simulink library "roller485lib"  (R2023a)
settings: Solver=VariableStepAuto  StartTime=0.0  StopTime=10.0  RelTol=1e-3
libraries: arduinolib x106, simulink x45
(part 2 of 3)

== system roller485lib/Basic I2C Write/position PID ==
  " x 10^5 " : Gain  Gain=1e5
  D : Constant  Value=position_D
  Data Type Conversion1 : DataTypeConversion  OutDataTypeStr=uint32  SaturateOnIntegerOverflow=off  RndMeth=Floor
  Data Type Conversion2 : DataTypeConversion  OutDataTypeStr=uint32  SaturateOnIntegerOverflow=off  RndMeth=Floor
  Data Type Conversion3 : DataTypeConversion  OutDataTypeStr=uint32  SaturateOnIntegerOverflow=off  RndMeth=Floor
  I : Constant  Value=position_I
  I2C Write (0xA0) : arduinolib/I2C Write  I2CModule=0  Mode=Master  SlaveAddress=I2CAddress  SlaveByteOrder=LittleEndian  Direction=Transmitter  RegisterAddressMode=on  RegisterAddress=0xA0  SlaveDataType=uint8  DataLength=1  NoAck=off  RepeatedStart=off  OutputStatus=off  blockPlatform=ARDUINO
  I2C Write (0xA4) : arduinolib/I2C Write  I2CModule=0  Mode=Master  SlaveAddress=I2CAddress  SlaveByteOrder=LittleEndian  Direction=Transmitter  RegisterAddressMode=on  RegisterAddress=0xA4  SlaveDataType=uint8  DataLength=1  NoAck=off  RepeatedStart=off  OutputStatus=off  blockPlatform=ARDUINO
  I2C Write (0xA8) : arduinolib/I2C Write  I2CModule=0  Mode=Master  SlaveAddress=I2CAddress  SlaveByteOrder=LittleEndian  Direction=Transmitter  RegisterAddressMode=on  RegisterAddress=0xA8  SlaveDataType=uint8  DataLength=1  NoAck=off  RepeatedStart=off  OutputStatus=off  blockPlatform=ARDUINO
  P : Constant  Value=position_P
  x 10^5 : Gain  Gain=1e5
  x 10^7 : Gain  Gain=1e7
  wires:
  P/1 -> x 10^5/1
  I/1 -> x 10^7/1
  D/1 -> " x 10^5 "/1
  Data Type Conversion1/1 -> I2C Write (0xA0)/1
  Data Type Conversion3/1 -> I2C Write (0xA8)/1
  Data Type Conversion2/1 -> I2C Write (0xA4)/1
  x 10^5/1 -> Data Type Conversion1/1
  x 10^7/1 -> Data Type Conversion2/1
  " x 10^5 "/1 -> Data Type Conversion3/1

== system roller485lib/Basic I2C Write/position PID (within set time) ==
  Clock : Clock
  Compare To Constant : simulink/Logic and Bit Operations/Compare To Constant  relop=<=  const=set_time  OutDataTypeStr=boolean
  D : Constant  Value=position_D
  Enabled Subsystem : Subsystem  TreatAsAtomicUnit=on
  I : Constant  Value=position_I
  P : Constant  Value=position_P
  wires:
  D/1 -> Enabled Subsystem/3(D)
  I/1 -> Enabled Subsystem/2(I)
  P/1 -> Enabled Subsystem/1(P)
  Compare To Constant/1 -> Enabled Subsystem/Enable
  Clock/1 -> Compare To Constant/1

== system roller485lib/Basic I2C Write/speed PID ==
  " x 10^5 " : Gain  Gain=1e5
  D : Constant  Value=speed_D
  Data Type Conversion2 : DataTypeConversion  OutDataTypeStr=uint32  SaturateOnIntegerOverflow=off  RndMeth=Floor
  Data Type Conversion4 : DataTypeConversion  OutDataTypeStr=uint32  SaturateOnIntegerOverflow=off  RndMeth=Floor
  Data Type Conversion6 : DataTypeConversion  OutDataTypeStr=uint32  SaturateOnIntegerOverflow=off  RndMeth=Floor
  I : Constant  Value=speed_I
  I2C Write (0x70) : arduinolib/I2C Write  I2CModule=0  Mode=Master  SlaveAddress=I2CAddress  SlaveByteOrder=LittleEndian  Direction=Transmitter  RegisterAddressMode=on  RegisterAddress=0x70  SlaveDataType=uint8  DataLength=1  NoAck=off  RepeatedStart=off  OutputStatus=off  blockPlatform=ARDUINO
  I2C Write (0x74) : arduinolib/I2C Write  I2CModule=0  Mode=Master  SlaveAddress=I2CAddress  SlaveByteOrder=LittleEndian  Direction=Transmitter  RegisterAddressMode=on  RegisterAddress=0x74  SlaveDataType=uint8  DataLength=1  NoAck=off  RepeatedStart=off  OutputStatus=off  blockPlatform=ARDUINO
  I2C Write (0x78) : arduinolib/I2C Write  I2CModule=0  Mode=Master  SlaveAddress=I2CAddress  SlaveByteOrder=LittleEndian  Direction=Transmitter  RegisterAddressMode=on  RegisterAddress=0x78  SlaveDataType=uint8  DataLength=1  NoAck=off  RepeatedStart=off  OutputStatus=off  blockPlatform=ARDUINO
  P : Constant  Value=speed_P
  x 10^5 : Gain  Gain=1e5
  x 10^7 : Gain  Gain=1e7
  wires:
  D/1 -> " x 10^5 "/1
  I/1 -> x 10^7/1
  P/1 -> x 10^5/1
  Data Type Conversion2/1 -> I2C Write (0x70)/1
  Data Type Conversion4/1 -> I2C Write (0x74)/1
  Data Type Conversion6/1 -> I2C Write (0x78)/1
  x 10^5/1 -> Data Type Conversion2/1
  x 10^7/1 -> Data Type Conversion4/1
  " x 10^5 "/1 -> Data Type Conversion6/1

== system roller485lib/Basic I2C Write/speed PID (within set time) ==
  Clock : Clock
  Compare To Constant : simulink/Logic and Bit Operations/Compare To Constant  relop=<=  const=set_time  OutDataTypeStr=boolean
  D : Constant  Value=speed_D
  Enabled Subsystem : Subsystem  TreatAsAtomicUnit=on
  I : Constant  Value=speed_I
  P : Constant  Value=speed_P
  wires:
  Clock/1 -> Compare To Constant/1
  Compare To Constant/1 -> Enabled Subsystem/Enable
  P/1 -> Enabled Subsystem/1(P)
  I/1 -> Enabled Subsystem/2(I)
  D/1 -> Enabled Subsystem/3(D)

== system roller485lib/I2C Read/absolute angle detection [deg] ==
  Data Type Conversion : DataTypeConversion  OutDataTypeStr=double  SaturateOnIntegerOverflow=off  RndMeth=Floor
  I2C Read (0x90) : arduinolib/I2C Read  I2CModule=0  Mode=Master  SlaveAddress=I2CAddress  SlaveByteOrder=LittleEndian  Direction=Receiver  RegisterAddressMode=on  RegisterAddress=0x90  SlaveDataType=int32  DataLength=1  NoAck=off  RepeatedStart=off  OutputStatus=off  blockPlatform=ARDUINO  SampleTime=sample_time
  Reshape : Reshape
  x (1/100) : Gain  Gain=1/100
  deg : Outport
  wires:
  x (1/100)/1 -> Reshape/1
  I2C Read (0x90)/1 -> Data Type Conversion/1
  Data Type Conversion/1 -> x (1/100)/1
  Reshape/1 -> deg/1

== system roller485lib/I2C Read/absolute angle detection [rad] ==
  Data Type Conversion : DataTypeConversion  OutDataTypeStr=double  SaturateOnIntegerOverflow=off  RndMeth=Floor
  I2C Read (0x90) : arduinolib/I2C Read  I2CModule=0  Mode=Master  SlaveAddress=I2CAddress  SlaveByteOrder=LittleEndian  Direction=Receiver  RegisterAddressMode=on  RegisterAddress=0x90  SlaveDataType=int32  DataLength=1  NoAck=off  RepeatedStart=off  OutputStatus=off  blockPlatform=ARDUINO  SampleTime=sample_time
  Reshape : Reshape
  deg to rad : Gain  Gain=pi/180
  x (1/100) : Gain  Gain=1/100
  rad : Outport
  wires:
  x (1/100)/1 -> deg to rad/1
  deg to rad/1 -> Reshape/1
  Data Type Conversion/1 -> x (1/100)/1
  I2C Read (0x90)/1 -> Data Type Conversion/1
  Reshape/1 -> rad/1

== system roller485lib/I2C Read/angular velocity detection using LPF [rad//s] ==
  Data Type Conversion : DataTypeConversion  OutDataTypeStr=double  SaturateOnIntegerOverflow=off  RndMeth=Floor
  I2C Read (0x60) : arduinolib/I2C Read  I2CModule=0  Mode=Master  SlaveAddress=I2CAddress  SlaveByteOrder=LittleEndian  Direction=Receiver  RegisterAddressMode=on  RegisterAddress=0x60  SlaveDataType=int32  DataLength=1  NoAck=off  RepeatedStart=off  OutputStatus=off  blockPlatform=ARDUINO  SampleTime=sample_time
  Reshape : Reshape
  rpm to rad/s : Gain  Gain=2*pi/60
  x (1/100) : Gain  Gain=1/100
  rad/s : Outport
  wires:
  x (1/100)/1 -> rpm to rad/s/1
  rpm to rad/s/1 -> Reshape/1
  I2C Read (0x60)/1 -> Data Type Conversion/1
  Data Type Conversion/1 -> x (1/100)/1
  Reshape/1 -> rad/s/1

== system roller485lib/I2C Read/angular velocity detection using LPF [rpm] ==
  Data Type Conversion : DataTypeConversion  OutDataTypeStr=double  SaturateOnIntegerOverflow=off  RndMeth=Floor
  I2C Read (0x60) : arduinolib/I2C Read  I2CModule=0  Mode=Master  SlaveAddress=I2CAddress  SlaveByteOrder=LittleEndian  Direction=Receiver  RegisterAddressMode=on  RegisterAddress=0x60  SlaveDataType=int32  DataLength=1  NoAck=off  RepeatedStart=off  OutputStatus=off  blockPlatform=ARDUINO  SampleTime=sample_time
  Reshape : Reshape
  x (1/100) : Gain  Gain=1/100
  rpm : Outport
  wires:
  x (1/100)/1 -> Reshape/1
  Data Type Conversion/1 -> x (1/100)/1
  I2C Read (0x60)/1 -> Data Type Conversion/1
  Reshape/1 -> rpm/1

== system roller485lib/I2C Read/current detection [A] ==
  Data Type Conversion : DataTypeConversion  OutDataTypeStr=double  SaturateOnIntegerOverflow=off  RndMeth=Floor
  I2C Read (0xC0) : arduinolib/I2C Read  I2CModule=0  Mode=Master  SlaveAddress=I2CAddress  SlaveByteOrder=LittleEndian  Direction=Receiver  RegisterAddressMode=on  RegisterAddress=0xC0  SlaveDataType=int32  DataLength=1  NoAck=off  RepeatedStart=off  OutputStatus=off  blockPlatform=ARDUINO  SampleTime=sample_time
  Reshape : Reshape
  mA to A : Gain  Gain=1/1000
  x (1/100) : Gain  Gain=1/100
  A : Outport
  wires:
  x (1/100)/1 -> mA to A/1
  Data Type Conversion/1 -> x (1/100)/1
  mA to A/1 -> Reshape/1
  I2C Read (0xC0)/1 -> Data Type Conversion/1
  Reshape/1 -> A/1

== system roller485lib/I2C Read/current detection [mA] ==
  Data Type Conversion : DataTypeConversion  OutDataTypeStr=double  SaturateOnIntegerOverflow=off  RndMeth=Floor
  I2C Read (0xC0) : arduinolib/I2C Read  I2CModule=0  Mode=Master  SlaveAddress=I2CAddress  SlaveByteOrder=LittleEndian  Direction=Receiver  RegisterAddressMode=on  RegisterAddress=0xC0  SlaveDataType=int32  DataLength=1  NoAck=off  RepeatedStart=off  OutputStatus=off  blockPlatform=ARDUINO  SampleTime=sample_time
  Reshape : Reshape
  x (1/100) : Gain  Gain=1/100
  mA : Outport
  wires:
  Data Type Conversion/1 -> x (1/100)/1
  x (1/100)/1 -> Reshape/1
  I2C Read (0xC0)/1 -> Data Type Conversion/1
  Reshape/1 -> mA/1

== system roller485lib/I2C Read/relative angle detection [deg] ==
  Clock : Clock
  Compare To Constant : simulink/Logic and Bit Operations/Compare To Constant  relop=<=  const=set_time  OutDataTypeStr=boolean
  Data Type Conversion : DataTypeConversion  OutDataTypeStr=double  SaturateOnIntegerOverflow=off  RndMeth=Floor
  Enabled Subsystem (initialization of angle) : Subsystem  TreatAsAtomicUnit=on
  I2C Read (0x90) : arduinolib/I2C Read  I2CModule=0  Mode=Master  SlaveAddress=I2CAddress  SlaveByteOrder=LittleEndian  Direction=Receiver  RegisterAddressMode=on  RegisterAddress=0x90  SlaveDataType=int32  DataLength=1  NoAck=off  RepeatedStart=off  OutputStatus=off  blockPlatform=ARDUINO  SampleTime=sample_time
  Reshape : Reshape
  Sum : Sum  Inputs=-+|
  x (1/100) : Gain  Gain=1/100
  deg : Outport
  wires:
  Sum/1 -> x (1/100)/1
  Enabled Subsystem (initialization of angle)/1(phim(0)) -> Sum/1
  Data Type Conversion/1 -> Sum/2, Enabled Subsystem (initialization of angle)/1(phim)
  Clock/1 -> Compare To Constant/1
  x (1/100)/1 -> Reshape/1
  I2C Read (0x90)/1 -> Data Type Conversion/1
  Reshape/1 -> deg/1
  Compare To Constant/1 -> Enabled Subsystem (initialization of angle)/Enable

== system roller485lib/I2C Read/relative angle detection [rad] ==
  Clock : Clock
  Compare To Constant : simulink/Logic and Bit Operations/Compare To Constant  relop=<=  const=set_time  OutDataTypeStr=boolean
  Data Type Conversion : DataTypeConversion  OutDataTypeStr=double  SaturateOnIntegerOverflow=off  RndMeth=Floor
  Enabled Subsystem (initialization of angle) : Subsystem  TreatAsAtomicUnit=on
  I2C Read (0x90) : arduinolib/I2C Read  I2CModule=0  Mode=Master  SlaveAddress=I2CAddress  SlaveByteOrder=LittleEndian  Direction=Receiver  RegisterAddressMode=on  RegisterAddress=0x90  SlaveDataType=int32  DataLength=1  NoAck=off  RepeatedStart=off  OutputStatus=off  blockPlatform=ARDUINO  SampleTime=sample_time
  Reshape : Reshape
  Sum : Sum  Inputs=-+|
  deg to rad : Gain  Gain=pi/180
  x (1/100) : Gain  Gain=1/100
  rad : Outport
  wires:
  x (1/100)/1 -> deg to rad/1
  Clock/1 -> Compare To Constant/1
  Data Type Conversion/1 -> Enabled Subsystem (initialization of angle)/1(phim), Sum/2
  Enabled Subsystem (initialization of angle)/1(phim(0)) -> Sum/1
  Sum/1 -> x (1/100)/1
  deg to rad/1 -> Reshape/1
  I2C Read (0x90)/1 -> Data Type Conversion/1
  Reshape/1 -> rad/1
  Compare To Constant/1 -> Enabled Subsystem (initialization of angle)/Enable

== system roller485lib/I2C Write/absolute angle command [deg] ==
  command [deg] : Inport
  Clock1 : Clock
  Clock2 : Clock
  Compare To Constant1 : simulink/Logic and Bit Operations/Compare To Constant  relop=<=  const=set_time1  OutDataTypeStr=boolean
  Compare To Constant2 : simulink/Logic and Bit Operations/Compare To Constant  relop=<=  const=set_time2  OutDataTypeStr=boolean
  D : Constant  Value=position_D
  Data Type Conversion : DataTypeConversion  OutDataTypeStr=uint32  SaturateOnIntegerOverflow=off  RndMeth=Floor
  Enabled Subsystem (PID setting) : Subsystem  TreatAsAtomicUnit=on
  Enabled Subsystem (mode setting) : Subsystem  TreatAsAtomicUnit=on
  I : Constant  Value=position_I
  I2C Write (0x80) : arduinolib/I2C Write  I2CModule=0  Mode=Master  SlaveAddress=I2CAddress  SlaveByteOrder=LittleEndian  Direction=Transmitter  RegisterAddressMode=on  RegisterAddress=0x80  SlaveDataType=uint8  DataLength=1  NoAck=off  RepeatedStart=off  OutputStatus=off  blockPlatform=ARDUINO
  P : Constant  Value=position_P
  position mode : Constant  Value=2
  x 100 : Gain  Gain=100
  wires:
  P/1 -> Enabled Subsystem (PID setting)/1(P)
  Clock1/1 -> Compare To Constant1/1
  position mode/1 -> Enabled Subsystem (mode setting)/1(mode)
  I/1 -> Enabled Subsystem (PID setting)/2(I)
  x 100/1 -> Data Type Conversion/1
  D/1 -> Enabled Subsystem (PID setting)/3(D)
  Compare To Constant2/1 -> Enabled Subsystem (PID setting)/Enable
  Compare To Constant1/1 -> Enabled Subsystem (mode setting)/Enable
  Clock2/1 -> Compare To Constant2/1
  Data Type Conversion/1 -> I2C Write (0x80)/1
  command [deg]/1 -> x 100/1

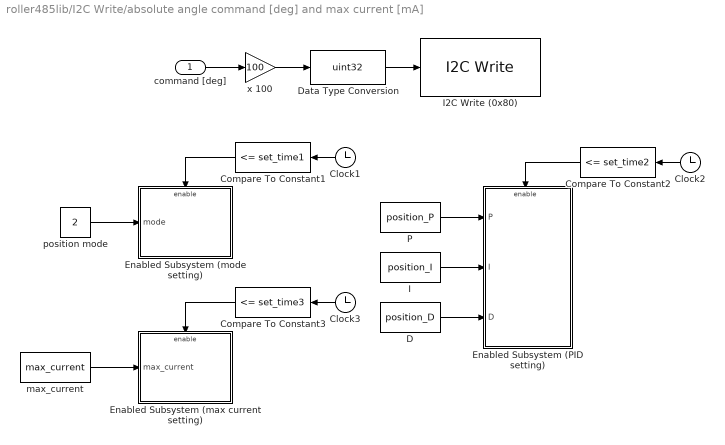
== system roller485lib/I2C Write/absolute angle command [deg] and max current [mA] ==
  command [deg] : Inport
  Clock1 : Clock
  Clock2 : Clock
  Clock3 : Clock
  Compare To Constant1 : simulink/Logic and Bit Operations/Compare To Constant  relop=<=  const=set_time1  OutDataTypeStr=boolean
  Compare To Constant2 : simulink/Logic and Bit Operations/Compare To Constant  relop=<=  const=set_time2  OutDataTypeStr=boolean
  Compare To Constant3 : simulink/Logic and Bit Operations/Compare To Constant  relop=<=  const=set_time3  OutDataTypeStr=boolean
  D : Constant  Value=position_D
  Data Type Conversion : DataTypeConversion  OutDataTypeStr=uint32  SaturateOnIntegerOverflow=off  RndMeth=Floor
  Enabled Subsystem (PID setting) : Subsystem  TreatAsAtomicUnit=on
  Enabled Subsystem (max current setting) : Subsystem  TreatAsAtomicUnit=on
  Enabled Subsystem (mode setting) : Subsystem  TreatAsAtomicUnit=on
  I : Constant  Value=position_I
  I2C Write (0x80) : arduinolib/I2C Write  I2CModule=0  Mode=Master  SlaveAddress=I2CAddress  SlaveByteOrder=LittleEndian  Direction=Transmitter  RegisterAddressMode=on  RegisterAddress=0x80  SlaveDataType=uint8  DataLength=1  NoAck=off  RepeatedStart=off  OutputStatus=off  blockPlatform=ARDUINO
  P : Constant  Value=position_P
  max_current : Constant  Value=max_current
  position mode : Constant  Value=2
  x 100 : Gain  Gain=100
  wires:
  P/1 -> Enabled Subsystem (PID setting)/1(P)
  Clock1/1 -> Compare To Constant1/1
  position mode/1 -> Enabled Subsystem (mode setting)/1(mode)
  I/1 -> Enabled Subsystem (PID setting)/2(I)
  Clock3/1 -> Compare To Constant3/1
  x 100/1 -> Data Type Conversion/1
  Compare To Constant3/1 -> Enabled Subsystem (max current setting)/Enable
  D/1 -> Enabled Subsystem (PID setting)/3(D)
  Compare To Constant2/1 -> Enabled Subsystem (PID setting)/Enable
  Compare To Constant1/1 -> Enabled Subsystem (mode setting)/Enable
  Clock2/1 -> Compare To Constant2/1
  max_current/1 -> Enabled Subsystem (max current setting)/1(max_current)
  Data Type Conversion/1 -> I2C Write (0x80)/1
  command [deg]/1 -> x 100/1

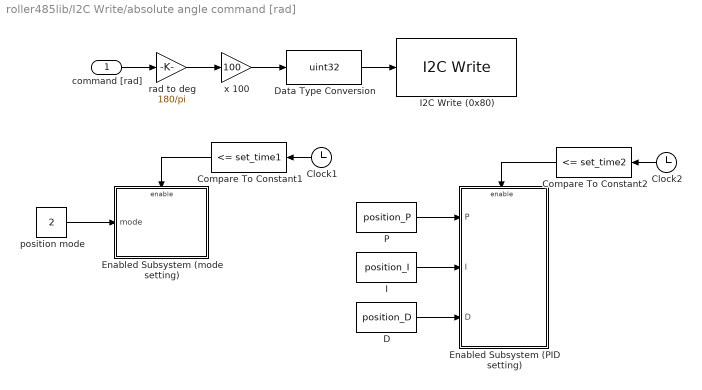
== system roller485lib/I2C Write/absolute angle command [rad] ==
  command [rad] : Inport
  Clock1 : Clock
  Clock2 : Clock
  Compare To Constant1 : simulink/Logic and Bit Operations/Compare To Constant  relop=<=  const=set_time1  OutDataTypeStr=boolean
  Compare To Constant2 : simulink/Logic and Bit Operations/Compare To Constant  relop=<=  const=set_time2  OutDataTypeStr=boolean
  D : Constant  Value=position_D
  Data Type Conversion : DataTypeConversion  OutDataTypeStr=uint32  SaturateOnIntegerOverflow=off  RndMeth=Floor
  Enabled Subsystem (PID setting) : Subsystem  TreatAsAtomicUnit=on
  Enabled Subsystem (mode setting) : Subsystem  TreatAsAtomicUnit=on
  I : Constant  Value=position_I
  I2C Write (0x80) : arduinolib/I2C Write  I2CModule=0  Mode=Master  SlaveAddress=I2CAddress  SlaveByteOrder=LittleEndian  Direction=Transmitter  RegisterAddressMode=on  RegisterAddress=0x80  SlaveDataType=uint8  DataLength=1  NoAck=off  RepeatedStart=off  OutputStatus=off  blockPlatform=ARDUINO
  P : Constant  Value=position_P
  position mode : Constant  Value=2
  rad to deg : Gain  Gain=180/pi
  x 100 : Gain  Gain=100
  wires:
  P/1 -> Enabled Subsystem (PID setting)/1(P)
  Clock1/1 -> Compare To Constant1/1
  position mode/1 -> Enabled Subsystem (mode setting)/1(mode)
  I/1 -> Enabled Subsystem (PID setting)/2(I)
  x 100/1 -> Data Type Conversion/1
  command [rad]/1 -> rad to deg/1
  D/1 -> Enabled Subsystem (PID setting)/3(D)
  Compare To Constant2/1 -> Enabled Subsystem (PID setting)/Enable
  Compare To Constant1/1 -> Enabled Subsystem (mode setting)/Enable
  Clock2/1 -> Compare To Constant2/1
  Data Type Conversion/1 -> I2C Write (0x80)/1
  rad to deg/1 -> x 100/1

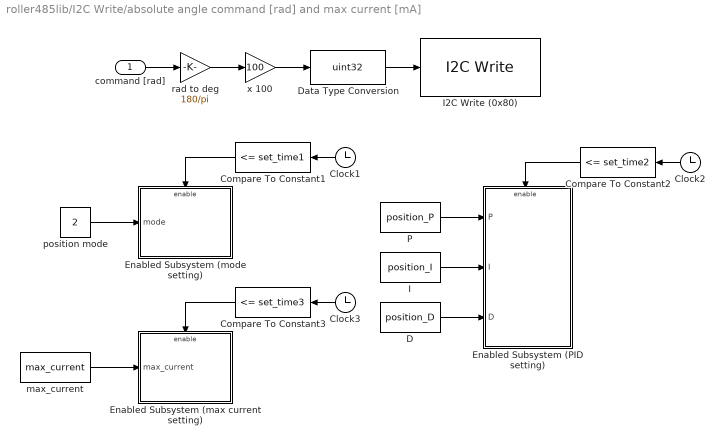
== system roller485lib/I2C Write/absolute angle command [rad] and max current [mA] ==
  command [rad] : Inport
  Clock1 : Clock
  Clock2 : Clock
  Clock3 : Clock
  Compare To Constant1 : simulink/Logic and Bit Operations/Compare To Constant  relop=<=  const=set_time1  OutDataTypeStr=boolean
  Compare To Constant2 : simulink/Logic and Bit Operations/Compare To Constant  relop=<=  const=set_time2  OutDataTypeStr=boolean
  Compare To Constant3 : simulink/Logic and Bit Operations/Compare To Constant  relop=<=  const=set_time3  OutDataTypeStr=boolean
  D : Constant  Value=position_D
  Data Type Conversion : DataTypeConversion  OutDataTypeStr=uint32  SaturateOnIntegerOverflow=off  RndMeth=Floor
  Enabled Subsystem (PID setting) : Subsystem  TreatAsAtomicUnit=on
  Enabled Subsystem (max current setting) : Subsystem  TreatAsAtomicUnit=on
  Enabled Subsystem (mode setting) : Subsystem  TreatAsAtomicUnit=on
  I : Constant  Value=position_I
  I2C Write (0x80) : arduinolib/I2C Write  I2CModule=0  Mode=Master  SlaveAddress=I2CAddress  SlaveByteOrder=LittleEndian  Direction=Transmitter  RegisterAddressMode=on  RegisterAddress=0x80  SlaveDataType=uint8  DataLength=1  NoAck=off  RepeatedStart=off  OutputStatus=off  blockPlatform=ARDUINO
  P : Constant  Value=position_P
  max_current : Constant  Value=max_current
  position mode : Constant  Value=2
  rad to deg : Gain  Gain=180/pi
  x 100 : Gain  Gain=100
  wires:
  command [rad]/1 -> rad to deg/1
  rad to deg/1 -> x 100/1
  Data Type Conversion/1 -> I2C Write (0x80)/1
  x 100/1 -> Data Type Conversion/1
  P/1 -> Enabled Subsystem (PID setting)/1(P)
  Clock1/1 -> Compare To Constant1/1
  Compare To Constant2/1 -> Enabled Subsystem (PID setting)/Enable
  I/1 -> Enabled Subsystem (PID setting)/2(I)
  D/1 -> Enabled Subsystem (PID setting)/3(D)
  Compare To Constant3/1 -> Enabled Subsystem (max current setting)/Enable
  Clock3/1 -> Compare To Constant3/1
  position mode/1 -> Enabled Subsystem (mode setting)/1(mode)
  max_current/1 -> Enabled Subsystem (max current setting)/1(max_current)
  Compare To Constant1/1 -> Enabled Subsystem (mode setting)/Enable
  Clock2/1 -> Compare To Constant2/1

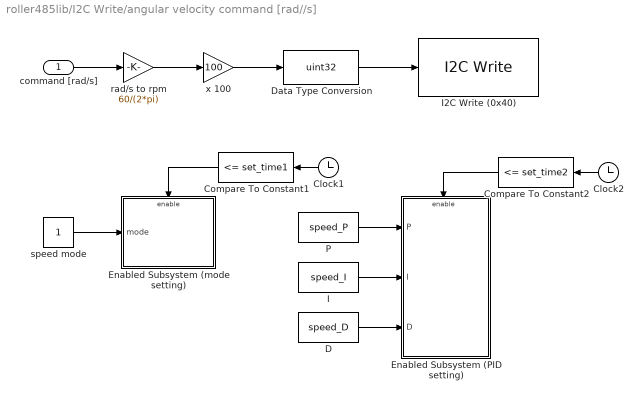
== system roller485lib/I2C Write/angular velocity command [rad//s] ==
  command [rad/s] : Inport
  Clock1 : Clock
  Clock2 : Clock
  Compare To Constant1 : simulink/Logic and Bit Operations/Compare To Constant  relop=<=  const=set_time1  OutDataTypeStr=boolean
  Compare To Constant2 : simulink/Logic and Bit Operations/Compare To Constant  relop=<=  const=set_time2  OutDataTypeStr=boolean
  D : Constant  Value=speed_D
  Data Type Conversion : DataTypeConversion  OutDataTypeStr=uint32  SaturateOnIntegerOverflow=off  RndMeth=Floor
  Enabled Subsystem (PID setting) : Subsystem  TreatAsAtomicUnit=on
  Enabled Subsystem (mode setting) : Subsystem  TreatAsAtomicUnit=on
  I : Constant  Value=speed_I
  I2C Write (0x40) : arduinolib/I2C Write  I2CModule=0  Mode=Master  SlaveAddress=I2CAddress  SlaveByteOrder=LittleEndian  Direction=Transmitter  RegisterAddressMode=on  RegisterAddress=0x40  SlaveDataType=uint8  DataLength=1  NoAck=off  RepeatedStart=off  OutputStatus=off  blockPlatform=ARDUINO
  P : Constant  Value=speed_P
  rad/s to rpm : Gain  Gain=60/(2*pi)
  speed mode : Constant
  x 100 : Gain  Gain=100
  wires:
  command [rad/s]/1 -> rad/s to rpm/1
  rad/s to rpm/1 -> x 100/1
  Data Type Conversion/1 -> I2C Write (0x40)/1
  I/1 -> Enabled Subsystem (PID setting)/2(I)
  P/1 -> Enabled Subsystem (PID setting)/1(P)
  speed mode/1 -> Enabled Subsystem (mode setting)/1(mode)
  D/1 -> Enabled Subsystem (PID setting)/3(D)
  x 100/1 -> Data Type Conversion/1
  Compare To Constant1/1 -> Enabled Subsystem (mode setting)/Enable
  Clock2/1 -> Compare To Constant2/1
  Clock1/1 -> Compare To Constant1/1
  Compare To Constant2/1 -> Enabled Subsystem (PID setting)/Enable

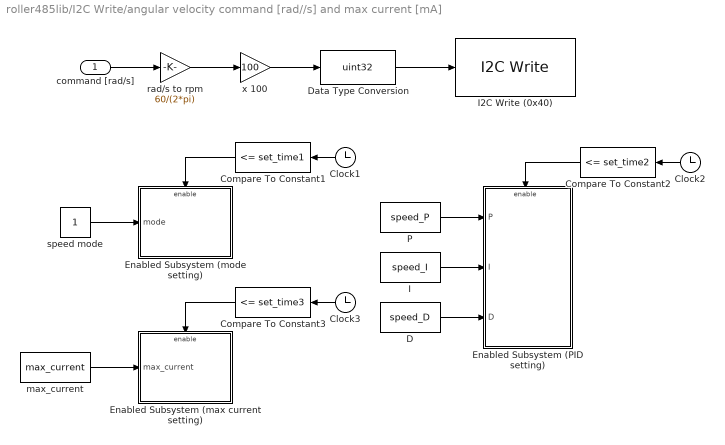
== system roller485lib/I2C Write/angular velocity command [rad//s] and max current [mA] ==
  command [rad/s] : Inport
  Clock1 : Clock
  Clock2 : Clock
  Clock3 : Clock
  Compare To Constant1 : simulink/Logic and Bit Operations/Compare To Constant  relop=<=  const=set_time1  OutDataTypeStr=boolean
  Compare To Constant2 : simulink/Logic and Bit Operations/Compare To Constant  relop=<=  const=set_time2  OutDataTypeStr=boolean
  Compare To Constant3 : simulink/Logic and Bit Operations/Compare To Constant  relop=<=  const=set_time3  OutDataTypeStr=boolean
  D : Constant  Value=speed_D
  Data Type Conversion : DataTypeConversion  OutDataTypeStr=uint32  SaturateOnIntegerOverflow=off  RndMeth=Floor
  Enabled Subsystem (PID setting) : Subsystem  TreatAsAtomicUnit=on
  Enabled Subsystem (max current setting) : Subsystem  TreatAsAtomicUnit=on
  Enabled Subsystem (mode setting) : Subsystem  TreatAsAtomicUnit=on
  I : Constant  Value=speed_I
  I2C Write (0x40) : arduinolib/I2C Write  I2CModule=0  Mode=Master  SlaveAddress=I2CAddress  SlaveByteOrder=LittleEndian  Direction=Transmitter  RegisterAddressMode=on  RegisterAddress=0x40  SlaveDataType=uint8  DataLength=1  NoAck=off  RepeatedStart=off  OutputStatus=off  blockPlatform=ARDUINO
  P : Constant  Value=speed_P
  max_current : Constant  Value=max_current
  rad/s to rpm : Gain  Gain=60/(2*pi)
  speed mode : Constant
  x 100 : Gain  Gain=100
  wires:
  command [rad/s]/1 -> rad/s to rpm/1
  rad/s to rpm/1 -> x 100/1
  Data Type Conversion/1 -> I2C Write (0x40)/1
  x 100/1 -> Data Type Conversion/1
  Clock2/1 -> Compare To Constant2/1
  Clock1/1 -> Compare To Constant1/1
  Clock3/1 -> Compare To Constant3/1
  Compare To Constant2/1 -> Enabled Subsystem (PID setting)/Enable
  D/1 -> Enabled Subsystem (PID setting)/3(D)
  I/1 -> Enabled Subsystem (PID setting)/2(I)
  P/1 -> Enabled Subsystem (PID setting)/1(P)
  max_current/1 -> Enabled Subsystem (max current setting)/1(max_current)
  speed mode/1 -> Enabled Subsystem (mode setting)/1(mode)
  Compare To Constant1/1 -> Enabled Subsystem (mode setting)/Enable
  Compare To Constant3/1 -> Enabled Subsystem (max current setting)/Enable

== system roller485lib/I2C Write/angular velocity command [rpm] ==
  command [rpm] : Inport
  Clock1 : Clock
  Clock2 : Clock
  Compare To Constant1 : simulink/Logic and Bit Operations/Compare To Constant  relop=<=  const=set_time1  OutDataTypeStr=boolean
  Compare To Constant2 : simulink/Logic and Bit Operations/Compare To Constant  relop=<=  const=set_time2  OutDataTypeStr=boolean
  D : Constant  Value=speed_D
  Data Type Conversion : DataTypeConversion  OutDataTypeStr=uint32  SaturateOnIntegerOverflow=off  RndMeth=Floor
  Enabled Subsystem (PID setting) : Subsystem  TreatAsAtomicUnit=on
  Enabled Subsystem (mode setting) : Subsystem  TreatAsAtomicUnit=on
  I : Constant  Value=speed_I
  I2C Write (0x40) : arduinolib/I2C Write  I2CModule=0  Mode=Master  SlaveAddress=I2CAddress  SlaveByteOrder=LittleEndian  Direction=Transmitter  RegisterAddressMode=on  RegisterAddress=0x40  SlaveDataType=uint8  DataLength=1  NoAck=off  RepeatedStart=off  OutputStatus=off  blockPlatform=ARDUINO
  P : Constant  Value=speed_P
  speed mode : Constant
  x 100 : Gain  Gain=100
  wires:
  Compare To Constant2/1 -> Enabled Subsystem (PID setting)/Enable
  Clock1/1 -> Compare To Constant1/1
  Clock2/1 -> Compare To Constant2/1
  Compare To Constant1/1 -> Enabled Subsystem (mode setting)/Enable
  x 100/1 -> Data Type Conversion/1
  D/1 -> Enabled Subsystem (PID setting)/3(D)
  speed mode/1 -> Enabled Subsystem (mode setting)/1(mode)
  P/1 -> Enabled Subsystem (PID setting)/1(P)
  I/1 -> Enabled Subsystem (PID setting)/2(I)
  Data Type Conversion/1 -> I2C Write (0x40)/1
  command [rpm]/1 -> x 100/1

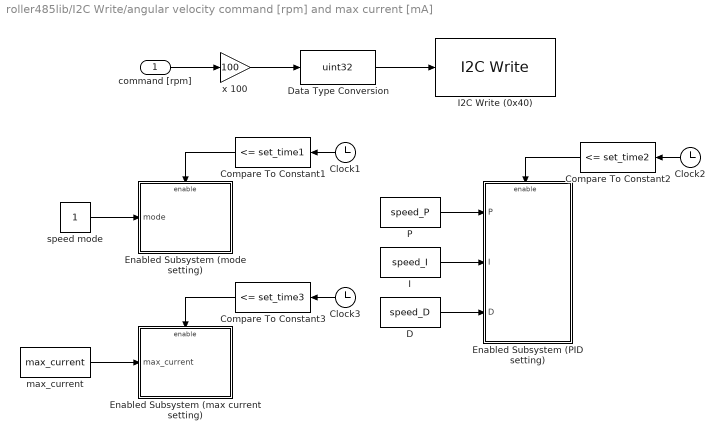
== system roller485lib/I2C Write/angular velocity command [rpm] and max current [mA] ==
  command [rpm] : Inport
  Clock1 : Clock
  Clock2 : Clock
  Clock3 : Clock
  Compare To Constant1 : simulink/Logic and Bit Operations/Compare To Constant  relop=<=  const=set_time1  OutDataTypeStr=boolean
  Compare To Constant2 : simulink/Logic and Bit Operations/Compare To Constant  relop=<=  const=set_time2  OutDataTypeStr=boolean
  Compare To Constant3 : simulink/Logic and Bit Operations/Compare To Constant  relop=<=  const=set_time3  OutDataTypeStr=boolean
  D : Constant  Value=speed_D
  Data Type Conversion : DataTypeConversion  OutDataTypeStr=uint32  SaturateOnIntegerOverflow=off  RndMeth=Floor
  Enabled Subsystem (PID setting) : Subsystem  TreatAsAtomicUnit=on
  Enabled Subsystem (max current setting) : Subsystem  TreatAsAtomicUnit=on
  Enabled Subsystem (mode setting) : Subsystem  TreatAsAtomicUnit=on
  I : Constant  Value=speed_I
  I2C Write (0x40) : arduinolib/I2C Write  I2CModule=0  Mode=Master  SlaveAddress=I2CAddress  SlaveByteOrder=LittleEndian  Direction=Transmitter  RegisterAddressMode=on  RegisterAddress=0x40  SlaveDataType=uint8  DataLength=1  NoAck=off  RepeatedStart=off  OutputStatus=off  blockPlatform=ARDUINO
  P : Constant  Value=speed_P
  max_current : Constant  Value=max_current
  speed mode : Constant
  x 100 : Gain  Gain=100
  wires:
  x 100/1 -> Data Type Conversion/1
  D/1 -> Enabled Subsystem (PID setting)/3(D)
  speed mode/1 -> Enabled Subsystem (mode setting)/1(mode)
  P/1 -> Enabled Subsystem (PID setting)/1(P)
  I/1 -> Enabled Subsystem (PID setting)/2(I)
  Data Type Conversion/1 -> I2C Write (0x40)/1
  command [rpm]/1 -> x 100/1
  max_current/1 -> Enabled Subsystem (max current setting)/1(max_current)
  Compare To Constant3/1 -> Enabled Subsystem (max current setting)/Enable
  Compare To Constant1/1 -> Enabled Subsystem (mode setting)/Enable
  Clock2/1 -> Compare To Constant2/1
  Clock1/1 -> Compare To Constant1/1
  Compare To Constant2/1 -> Enabled Subsystem (PID setting)/Enable
  Clock3/1 -> Compare To Constant3/1

== system roller485lib/I2C Write/current command [A] ==
  command [A] : Inport
  A to mA : Gain  Gain=1000
  "Clock " : Clock
  Compare To Constant : simulink/Logic and Bit Operations/Compare To Constant  relop=<=  const=set_time  OutDataTypeStr=boolean
  Data Type Conversion : DataTypeConversion  OutDataTypeStr=uint32  SaturateOnIntegerOverflow=off  RndMeth=Floor
  Enabled Subsystem (mode setting) : Subsystem  TreatAsAtomicUnit=on
  I2C Write (0xB0) : arduinolib/I2C Write  I2CModule=0  Mode=Master  SlaveAddress=I2CAddress  SlaveByteOrder=LittleEndian  Direction=Transmitter  RegisterAddressMode=on  RegisterAddress=0xB0  SlaveDataType=uint8  DataLength=1  NoAck=off  RepeatedStart=off  OutputStatus=off  blockPlatform=ARDUINO
  current mode : Constant  Value=3
  x 100 : Gain  Gain=100
  wires:
  x 100/1 -> Data Type Conversion/1
  command [A]/1 -> A to mA/1
  Data Type Conversion/1 -> I2C Write (0xB0)/1
  "Clock "/1 -> Compare To Constant/1
  Compare To Constant/1 -> Enabled Subsystem (mode setting)/Enable
  current mode/1 -> Enabled Subsystem (mode setting)/1(mode)
  A to mA/1 -> x 100/1

== system roller485lib/I2C Write/current command [mA] ==
  command [mA] : Inport
  "Clock " : Clock
  Compare To Constant : simulink/Logic and Bit Operations/Compare To Constant  relop=<=  const=set_time  OutDataTypeStr=boolean
  Data Type Conversion : DataTypeConversion  OutDataTypeStr=uint32  SaturateOnIntegerOverflow=off  RndMeth=Floor
  Enabled Subsystem (mode setting) : Subsystem  TreatAsAtomicUnit=on
  I2C Write (0xB0) : arduinolib/I2C Write  I2CModule=0  Mode=Master  SlaveAddress=I2CAddress  SlaveByteOrder=LittleEndian  Direction=Transmitter  RegisterAddressMode=on  RegisterAddress=0xB0  SlaveDataType=uint8  DataLength=1  NoAck=off  RepeatedStart=off  OutputStatus=off  blockPlatform=ARDUINO
  current mode : Constant  Value=3
  x 100 : Gain  Gain=100
  wires:
  current mode/1 -> Enabled Subsystem (mode setting)/1(mode)
  Compare To Constant/1 -> Enabled Subsystem (mode setting)/Enable
  "Clock "/1 -> Compare To Constant/1
  Data Type Conversion/1 -> I2C Write (0xB0)/1
  command [mA]/1 -> x 100/1
  x 100/1 -> Data Type Conversion/1

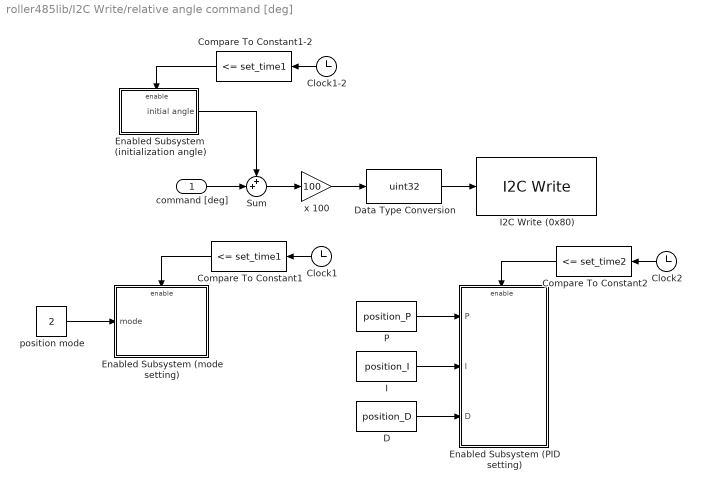
== system roller485lib/I2C Write/relative angle command [deg] ==
  command [deg] : Inport
  Clock1 : Clock
  Clock1-2 : Clock
  Clock2 : Clock
  Compare To Constant1 : simulink/Logic and Bit Operations/Compare To Constant  relop=<=  const=set_time1  OutDataTypeStr=boolean
  Compare To Constant1-2 : simulink/Logic and Bit Operations/Compare To Constant  relop=<=  const=set_time1  OutDataTypeStr=boolean
  Compare To Constant2 : simulink/Logic and Bit Operations/Compare To Constant  relop=<=  const=set_time2  OutDataTypeStr=boolean
  D : Constant  Value=position_D
  Data Type Conversion : DataTypeConversion  OutDataTypeStr=uint32  SaturateOnIntegerOverflow=off  RndMeth=Floor
  Enabled Subsystem (PID setting) : Subsystem  TreatAsAtomicUnit=on
  Enabled Subsystem (initialization angle) : Subsystem  TreatAsAtomicUnit=on
  Enabled Subsystem (mode setting) : Subsystem  TreatAsAtomicUnit=on
  I : Constant  Value=position_I
  I2C Write (0x80) : arduinolib/I2C Write  I2CModule=0  Mode=Master  SlaveAddress=I2CAddress  SlaveByteOrder=LittleEndian  Direction=Transmitter  RegisterAddressMode=on  RegisterAddress=0x80  SlaveDataType=uint8  DataLength=1  NoAck=off  RepeatedStart=off  OutputStatus=off  blockPlatform=ARDUINO
  P : Constant  Value=position_P
  Sum : Sum  Inputs=++|
  position mode : Constant  Value=2
  x 100 : Gain  Gain=100
  wires:
  Compare To Constant1-2/1 -> Enabled Subsystem (initialization angle)/Enable
  command [deg]/1 -> Sum/2
  Enabled Subsystem (initialization angle)/1(initial angle) -> Sum/1
  x 100/1 -> Data Type Conversion/1
  Sum/1 -> x 100/1
  Compare To Constant2/1 -> Enabled Subsystem (PID setting)/Enable
  position mode/1 -> Enabled Subsystem (mode setting)/1(mode)
  P/1 -> Enabled Subsystem (PID setting)/1(P)
  Clock1/1 -> Compare To Constant1/1
  Compare To Constant1/1 -> Enabled Subsystem (mode setting)/Enable
  Data Type Conversion/1 -> I2C Write (0x80)/1
  D/1 -> Enabled Subsystem (PID setting)/3(D)
  I/1 -> Enabled Subsystem (PID setting)/2(I)
  Clock2/1 -> Compare To Constant2/1
  Clock1-2/1 -> Compare To Constant1-2/1

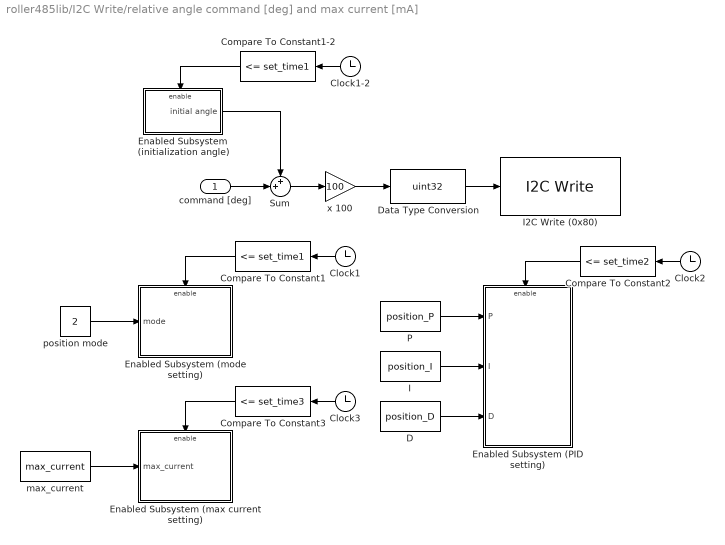
== system roller485lib/I2C Write/relative angle command [deg] and max current [mA] ==
  command [deg] : Inport
  Clock1 : Clock
  Clock1-2 : Clock
  Clock2 : Clock
  Clock3 : Clock
  Compare To Constant1 : simulink/Logic and Bit Operations/Compare To Constant  relop=<=  const=set_time1  OutDataTypeStr=boolean
  Compare To Constant1-2 : simulink/Logic and Bit Operations/Compare To Constant  relop=<=  const=set_time1  OutDataTypeStr=boolean
  Compare To Constant2 : simulink/Logic and Bit Operations/Compare To Constant  relop=<=  const=set_time2  OutDataTypeStr=boolean
  Compare To Constant3 : simulink/Logic and Bit Operations/Compare To Constant  relop=<=  const=set_time3  OutDataTypeStr=boolean
  D : Constant  Value=position_D
  Data Type Conversion : DataTypeConversion  OutDataTypeStr=uint32  SaturateOnIntegerOverflow=off  RndMeth=Floor
  Enabled Subsystem (PID setting) : Subsystem  TreatAsAtomicUnit=on
  Enabled Subsystem (initialization angle) : Subsystem  TreatAsAtomicUnit=on
  Enabled Subsystem (max current setting) : Subsystem  TreatAsAtomicUnit=on
  Enabled Subsystem (mode setting) : Subsystem  TreatAsAtomicUnit=on
  I : Constant  Value=position_I
  I2C Write (0x80) : arduinolib/I2C Write  I2CModule=0  Mode=Master  SlaveAddress=I2CAddress  SlaveByteOrder=LittleEndian  Direction=Transmitter  RegisterAddressMode=on  RegisterAddress=0x80  SlaveDataType=uint8  DataLength=1  NoAck=off  RepeatedStart=off  OutputStatus=off  blockPlatform=ARDUINO
  P : Constant  Value=position_P
  Sum : Sum  Inputs=++|
  max_current : Constant  Value=max_current
  position mode : Constant  Value=2
  x 100 : Gain  Gain=100
  wires:
  Compare To Constant1-2/1 -> Enabled Subsystem (initialization angle)/Enable
  command [deg]/1 -> Sum/2
  Enabled Subsystem (initialization angle)/1(initial angle) -> Sum/1
  x 100/1 -> Data Type Conversion/1
  Sum/1 -> x 100/1
  max_current/1 -> Enabled Subsystem (max current setting)/1(max_current)
  Compare To Constant2/1 -> Enabled Subsystem (PID setting)/Enable
  Compare To Constant3/1 -> Enabled Subsystem (max current setting)/Enable
  position mode/1 -> Enabled Subsystem (mode setting)/1(mode)
  P/1 -> Enabled Subsystem (PID setting)/1(P)
  Clock1/1 -> Compare To Constant1/1
  Compare To Constant1/1 -> Enabled Subsystem (mode setting)/Enable
  Data Type Conversion/1 -> I2C Write (0x80)/1
  D/1 -> Enabled Subsystem (PID setting)/3(D)
  I/1 -> Enabled Subsystem (PID setting)/2(I)
  Clock3/1 -> Compare To Constant3/1
  Clock2/1 -> Compare To Constant2/1
  Clock1-2/1 -> Compare To Constant1-2/1

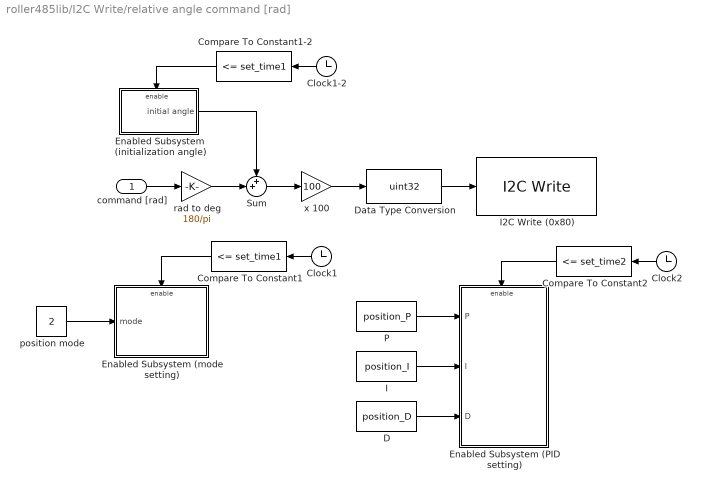
== system roller485lib/I2C Write/relative angle command [rad] ==
  command [rad] : Inport
  Clock1 : Clock
  Clock1-2 : Clock
  Clock2 : Clock
  Compare To Constant1 : simulink/Logic and Bit Operations/Compare To Constant  relop=<=  const=set_time1  OutDataTypeStr=boolean
  Compare To Constant1-2 : simulink/Logic and Bit Operations/Compare To Constant  relop=<=  const=set_time1  OutDataTypeStr=boolean
  Compare To Constant2 : simulink/Logic and Bit Operations/Compare To Constant  relop=<=  const=set_time2  OutDataTypeStr=boolean
  D : Constant  Value=position_D
  Data Type Conversion : DataTypeConversion  OutDataTypeStr=uint32  SaturateOnIntegerOverflow=off  RndMeth=Floor
  Enabled Subsystem (PID setting) : Subsystem  TreatAsAtomicUnit=on
  Enabled Subsystem (initialization angle) : Subsystem  TreatAsAtomicUnit=on
  Enabled Subsystem (mode setting) : Subsystem  TreatAsAtomicUnit=on
  I : Constant  Value=position_I
  I2C Write (0x80) : arduinolib/I2C Write  I2CModule=0  Mode=Master  SlaveAddress=I2CAddress  SlaveByteOrder=LittleEndian  Direction=Transmitter  RegisterAddressMode=on  RegisterAddress=0x80  SlaveDataType=uint8  DataLength=1  NoAck=off  RepeatedStart=off  OutputStatus=off  blockPlatform=ARDUINO
  P : Constant  Value=position_P
  Sum : Sum  Inputs=++|
  position mode : Constant  Value=2
  rad to deg : Gain  Gain=180/pi
  x 100 : Gain  Gain=100
  wires:
  Compare To Constant1-2/1 -> Enabled Subsystem (initialization angle)/Enable
  command [rad]/1 -> rad to deg/1
  rad to deg/1 -> Sum/2
  Enabled Subsystem (initialization angle)/1(initial angle) -> Sum/1
  x 100/1 -> Data Type Conversion/1
  Sum/1 -> x 100/1
  Compare To Constant2/1 -> Enabled Subsystem (PID setting)/Enable
  position mode/1 -> Enabled Subsystem (mode setting)/1(mode)
  P/1 -> Enabled Subsystem (PID setting)/1(P)
  Clock1/1 -> Compare To Constant1/1
  Compare To Constant1/1 -> Enabled Subsystem (mode setting)/Enable
  Data Type Conversion/1 -> I2C Write (0x80)/1
  D/1 -> Enabled Subsystem (PID setting)/3(D)
  I/1 -> Enabled Subsystem (PID setting)/2(I)
  Clock2/1 -> Compare To Constant2/1
  Clock1-2/1 -> Compare To Constant1-2/1

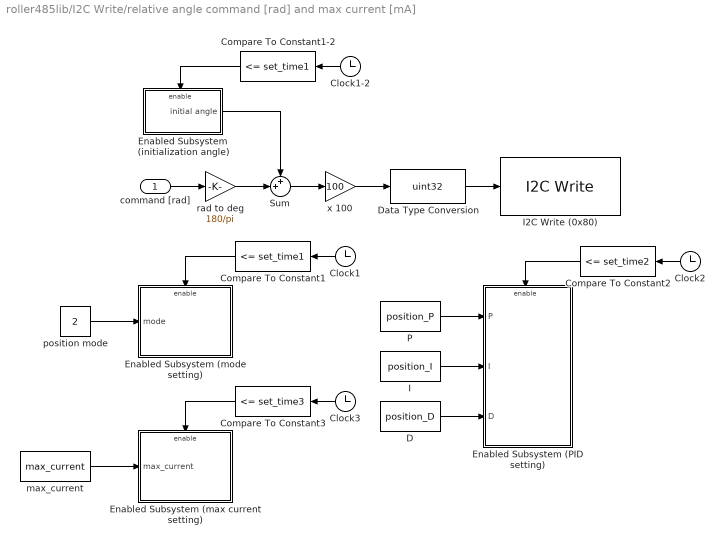
== system roller485lib/I2C Write/relative angle command [rad] and max current [mA] ==
  command [rad] : Inport
  Clock1 : Clock
  Clock1-2 : Clock
  Clock2 : Clock
  Clock3 : Clock
  Compare To Constant1 : simulink/Logic and Bit Operations/Compare To Constant  relop=<=  const=set_time1  OutDataTypeStr=boolean
  Compare To Constant1-2 : simulink/Logic and Bit Operations/Compare To Constant  relop=<=  const=set_time1  OutDataTypeStr=boolean
  Compare To Constant2 : simulink/Logic and Bit Operations/Compare To Constant  relop=<=  const=set_time2  OutDataTypeStr=boolean
  Compare To Constant3 : simulink/Logic and Bit Operations/Compare To Constant  relop=<=  const=set_time3  OutDataTypeStr=boolean
  D : Constant  Value=position_D
  Data Type Conversion : DataTypeConversion  OutDataTypeStr=uint32  SaturateOnIntegerOverflow=off  RndMeth=Floor
  Enabled Subsystem (PID setting) : Subsystem  TreatAsAtomicUnit=on
  Enabled Subsystem (initialization angle) : Subsystem  TreatAsAtomicUnit=on
  Enabled Subsystem (max current setting) : Subsystem  TreatAsAtomicUnit=on
  Enabled Subsystem (mode setting) : Subsystem  TreatAsAtomicUnit=on
  I : Constant  Value=position_I
  I2C Write (0x80) : arduinolib/I2C Write  I2CModule=0  Mode=Master  SlaveAddress=I2CAddress  SlaveByteOrder=LittleEndian  Direction=Transmitter  RegisterAddressMode=on  RegisterAddress=0x80  SlaveDataType=uint8  DataLength=1  NoAck=off  RepeatedStart=off  OutputStatus=off  blockPlatform=ARDUINO
  P : Constant  Value=position_P
  Sum : Sum  Inputs=++|
  max_current : Constant  Value=max_current
  position mode : Constant  Value=2
  rad to deg : Gain  Gain=180/pi
  x 100 : Gain  Gain=100
  wires:
  Enabled Subsystem (initialization angle)/1(initial angle) -> Sum/1
  command [rad]/1 -> rad to deg/1
  x 100/1 -> Data Type Conversion/1
  Sum/1 -> x 100/1
  Data Type Conversion/1 -> I2C Write (0x80)/1
  rad to deg/1 -> Sum/2
  Clock2/1 -> Compare To Constant2/1
  D/1 -> Enabled Subsystem (PID setting)/3(D)
  Compare To Constant1/1 -> Enabled Subsystem (mode setting)/Enable
  I/1 -> Enabled Subsystem (PID setting)/2(I)
  Clock1/1 -> Compare To Constant1/1
  position mode/1 -> Enabled Subsystem (mode setting)/1(mode)
  Compare To Constant3/1 -> Enabled Subsystem (max current setting)/Enable
  Clock3/1 -> Compare To Constant3/1
  P/1 -> Enabled Subsystem (PID setting)/1(P)
  max_current/1 -> Enabled Subsystem (max current setting)/1(max_current)
  Compare To Constant2/1 -> Enabled Subsystem (PID setting)/Enable
  Compare To Constant1-2/1 -> Enabled Subsystem (initialization angle)/Enable
  Clock1-2/1 -> Compare To Constant1-2/1

== system roller485lib/motor ON//OFF/Enabled Subsystem ==
  ON (1) or OFF (0) : Inport
  Enable : EnablePort
  Data Type Conversion : DataTypeConversion  OutDataTypeStr=uint8  SaturateOnIntegerOverflow=off  RndMeth=Floor
  I2C Write (0x00) : arduinolib/I2C Write  I2CModule=0  Mode=Master  SlaveAddress=I2CAddress  SlaveByteOrder=BigEndian  Direction=Transmitter  RegisterAddressMode=on  RegisterAddress=0x00  SlaveDataType=uint8  DataLength=1  NoAck=off  RepeatedStart=off  OutputStatus=off  blockPlatform=ARDUINO
  wires:
  ON (1) or OFF (0)/1 -> Data Type Conversion/1
  Data Type Conversion/1 -> I2C Write (0x00)/1

== system roller485lib/Basic I2C Write/basic relative angle command [deg]/Enabled Subsystem (initialization angle) ==
  Enable : EnablePort
  Data Type Conversion : DataTypeConversion  OutDataTypeStr=double  SaturateOnIntegerOverflow=off  RndMeth=Floor
  I2C Read (0x90) : arduinolib/I2C Read  I2CModule=0  Mode=Master  SlaveAddress=I2CAddress  SlaveByteOrder=LittleEndian  Direction=Receiver  RegisterAddressMode=on  RegisterAddress=0x90  SlaveDataType=int32  DataLength=1  NoAck=off  RepeatedStart=off  OutputStatus=off  blockPlatform=ARDUINO  SampleTime=sample_time
  x (1/100) : Gain  Gain=1/100
  initial angle : Outport
  wires:
  I2C Read (0x90)/1 -> Data Type Conversion/1
  Data Type Conversion/1 -> x (1/100)/1
  x (1/100)/1 -> initial angle/1

== system roller485lib/Basic I2C Write/basic relative angle command [rad]/Enabled Subsystem (initialization angle) ==
  Enable : EnablePort
  Data Type Conversion : DataTypeConversion  OutDataTypeStr=double  SaturateOnIntegerOverflow=off  RndMeth=Floor
  I2C Read (0x90) : arduinolib/I2C Read  I2CModule=0  Mode=Master  SlaveAddress=I2CAddress  SlaveByteOrder=LittleEndian  Direction=Receiver  RegisterAddressMode=on  RegisterAddress=0x90  SlaveDataType=int32  DataLength=1  NoAck=off  RepeatedStart=off  OutputStatus=off  blockPlatform=ARDUINO  SampleTime=sample_time
  x (1/100) : Gain  Gain=1/100
  initial angle : Outport
  wires:
  I2C Read (0x90)/1 -> Data Type Conversion/1
  Data Type Conversion/1 -> x (1/100)/1
  x (1/100)/1 -> initial angle/1

== system roller485lib/Basic I2C Write/control mode/Enabled Subsystem ==
  mode : Inport
  Enable : EnablePort
  Data Type Conversion : DataTypeConversion  OutDataTypeStr=uint8  SaturateOnIntegerOverflow=off  RndMeth=Floor
  I2C Write (0x01) : arduinolib/I2C Write  I2CModule=0  Mode=Master  SlaveAddress=I2CAddress  SlaveByteOrder=BigEndian  Direction=Transmitter  RegisterAddressMode=on  RegisterAddress=0x01  SlaveDataType=uint8  DataLength=1  NoAck=off  RepeatedStart=off  OutputStatus=off  blockPlatform=ARDUINO
  wires:
  Data Type Conversion/1 -> I2C Write (0x01)/1
  mode/1 -> Data Type Conversion/1

== system roller485lib/Basic I2C Write/position PID (within set time)/Enabled Subsystem ==
  P : Inport
  I : Inport  Port=2
  D : Inport  Port=3
  Enable : EnablePort
  " x 10^5 " : Gain  Gain=1e5
  Data Type Conversion1 : DataTypeConversion  OutDataTypeStr=uint32  SaturateOnIntegerOverflow=off  RndMeth=Floor
  Data Type Conversion2 : DataTypeConversion  OutDataTypeStr=uint32  SaturateOnIntegerOverflow=off  RndMeth=Floor
  Data Type Conversion3 : DataTypeConversion  OutDataTypeStr=uint32  SaturateOnIntegerOverflow=off  RndMeth=Floor
  I2C Write (0xA0) : arduinolib/I2C Write  I2CModule=0  Mode=Master  SlaveAddress=I2CAddress  SlaveByteOrder=LittleEndian  Direction=Transmitter  RegisterAddressMode=on  RegisterAddress=0xA0  SlaveDataType=uint8  DataLength=1  NoAck=off  RepeatedStart=off  OutputStatus=off  blockPlatform=ARDUINO
  I2C Write (0xA4) : arduinolib/I2C Write  I2CModule=0  Mode=Master  SlaveAddress=I2CAddress  SlaveByteOrder=LittleEndian  Direction=Transmitter  RegisterAddressMode=on  RegisterAddress=0xA4  SlaveDataType=uint8  DataLength=1  NoAck=off  RepeatedStart=off  OutputStatus=off  blockPlatform=ARDUINO
  I2C Write (0xA8) : arduinolib/I2C Write  I2CModule=0  Mode=Master  SlaveAddress=I2CAddress  SlaveByteOrder=LittleEndian  Direction=Transmitter  RegisterAddressMode=on  RegisterAddress=0xA8  SlaveDataType=uint8  DataLength=1  NoAck=off  RepeatedStart=off  OutputStatus=off  blockPlatform=ARDUINO
  x 10^5 : Gain  Gain=1e5
  x 10^7 : Gain  Gain=1e7
  wires:
  P/1 -> x 10^5/1
  I/1 -> x 10^7/1
  D/1 -> " x 10^5 "/1
  x 10^5/1 -> Data Type Conversion1/1
  x 10^7/1 -> Data Type Conversion2/1
  " x 10^5 "/1 -> Data Type Conversion3/1
  Data Type Conversion3/1 -> I2C Write (0xA8)/1
  Data Type Conversion2/1 -> I2C Write (0xA4)/1
  Data Type Conversion1/1 -> I2C Write (0xA0)/1

== system roller485lib/Basic I2C Write/speed PID (within set time)/Enabled Subsystem ==
  P : Inport
  I : Inport  Port=2
  D : Inport  Port=3
  Enable : EnablePort
  " x 10^5 " : Gain  Gain=1e5
  Data Type Conversion1 : DataTypeConversion  OutDataTypeStr=uint32  SaturateOnIntegerOverflow=off  RndMeth=Floor
  Data Type Conversion2 : DataTypeConversion  OutDataTypeStr=uint32  SaturateOnIntegerOverflow=off  RndMeth=Floor
  Data Type Conversion3 : DataTypeConversion  OutDataTypeStr=uint32  SaturateOnIntegerOverflow=off  RndMeth=Floor
  I2C Write (0x70) : arduinolib/I2C Write  I2CModule=0  Mode=Master  SlaveAddress=I2CAddress  SlaveByteOrder=LittleEndian  Direction=Transmitter  RegisterAddressMode=on  RegisterAddress=0x70  SlaveDataType=uint8  DataLength=1  NoAck=off  RepeatedStart=off  OutputStatus=off  blockPlatform=ARDUINO
  I2C Write (0x74) : arduinolib/I2C Write  I2CModule=0  Mode=Master  SlaveAddress=I2CAddress  SlaveByteOrder=LittleEndian  Direction=Transmitter  RegisterAddressMode=on  RegisterAddress=0x74  SlaveDataType=uint8  DataLength=1  NoAck=off  RepeatedStart=off  OutputStatus=off  blockPlatform=ARDUINO
  I2C Write (0x78) : arduinolib/I2C Write  I2CModule=0  Mode=Master  SlaveAddress=I2CAddress  SlaveByteOrder=LittleEndian  Direction=Transmitter  RegisterAddressMode=on  RegisterAddress=0x78  SlaveDataType=uint8  DataLength=1  NoAck=off  RepeatedStart=off  OutputStatus=off  blockPlatform=ARDUINO
  x 10^5 : Gain  Gain=1e5
  x 10^7 : Gain  Gain=1e7
  wires:
  D/1 -> " x 10^5 "/1
  I/1 -> x 10^7/1
  P/1 -> x 10^5/1
  x 10^5/1 -> Data Type Conversion1/1
  " x 10^5 "/1 -> Data Type Conversion3/1
  x 10^7/1 -> Data Type Conversion2/1
  Data Type Conversion2/1 -> I2C Write (0x74)/1
  Data Type Conversion3/1 -> I2C Write (0x78)/1
  Data Type Conversion1/1 -> I2C Write (0x70)/1

== system roller485lib/I2C Read/relative angle detection [deg]/Enabled Subsystem (initialization of angle) ==
  phim : Inport
  Enable : EnablePort
  phim(0) : Outport
  wires:
  phim/1 -> phim(0)/1

== system roller485lib/I2C Read/relative angle detection [rad]/Enabled Subsystem (initialization of angle) ==
  phim : Inport
  Enable : EnablePort
  phim(0) : Outport
  wires:
  phim/1 -> phim(0)/1

== system roller485lib/I2C Write/absolute angle command [deg]/Enabled Subsystem (PID setting) ==
  P : Inport
  I : Inport  Port=2
  D : Inport  Port=3
  Enable : EnablePort
  " x 10^5 " : Gain  Gain=1e5
  Data Type Conversion1 : DataTypeConversion  OutDataTypeStr=uint32  SaturateOnIntegerOverflow=off  RndMeth=Floor
  Data Type Conversion2 : DataTypeConversion  OutDataTypeStr=uint32  SaturateOnIntegerOverflow=off  RndMeth=Floor
  Data Type Conversion3 : DataTypeConversion  OutDataTypeStr=uint32  SaturateOnIntegerOverflow=off  RndMeth=Floor
  I2C Write (0xA0) : arduinolib/I2C Write  I2CModule=0  Mode=Master  SlaveAddress=I2CAddress  SlaveByteOrder=LittleEndian  Direction=Transmitter  RegisterAddressMode=on  RegisterAddress=0xA0  SlaveDataType=uint8  DataLength=1  NoAck=off  RepeatedStart=off  OutputStatus=off  blockPlatform=ARDUINO
  I2C Write (0xA4) : arduinolib/I2C Write  I2CModule=0  Mode=Master  SlaveAddress=I2CAddress  SlaveByteOrder=LittleEndian  Direction=Transmitter  RegisterAddressMode=on  RegisterAddress=0xA4  SlaveDataType=uint8  DataLength=1  NoAck=off  RepeatedStart=off  OutputStatus=off  blockPlatform=ARDUINO
  I2C Write (0xA8) : arduinolib/I2C Write  I2CModule=0  Mode=Master  SlaveAddress=I2CAddress  SlaveByteOrder=LittleEndian  Direction=Transmitter  RegisterAddressMode=on  RegisterAddress=0xA8  SlaveDataType=uint8  DataLength=1  NoAck=off  RepeatedStart=off  OutputStatus=off  blockPlatform=ARDUINO
  x 10^5 : Gain  Gain=1e5
  x 10^7 : Gain  Gain=1e7
  wires:
  P/1 -> x 10^5/1
  I/1 -> x 10^7/1
  D/1 -> " x 10^5 "/1
  Data Type Conversion2/1 -> I2C Write (0xA4)/1
  Data Type Conversion3/1 -> I2C Write (0xA8)/1
  Data Type Conversion1/1 -> I2C Write (0xA0)/1
  x 10^5/1 -> Data Type Conversion1/1
  x 10^7/1 -> Data Type Conversion2/1
  " x 10^5 "/1 -> Data Type Conversion3/1

== system roller485lib/I2C Write/absolute angle command [deg]/Enabled Subsystem (mode setting) ==
  mode : Inport
  Enable : EnablePort
  Data Type Conversion : DataTypeConversion  OutDataTypeStr=uint8  SaturateOnIntegerOverflow=off  RndMeth=Floor
  I2C Write (0x01) : arduinolib/I2C Write  I2CModule=0  Mode=Master  SlaveAddress=I2CAddress  SlaveByteOrder=BigEndian  Direction=Transmitter  RegisterAddressMode=on  RegisterAddress=0x01  SlaveDataType=uint8  DataLength=1  NoAck=off  RepeatedStart=off  OutputStatus=off  blockPlatform=ARDUINO
  wires:
  Data Type Conversion/1 -> I2C Write (0x01)/1
  mode/1 -> Data Type Conversion/1

== system roller485lib/I2C Write/absolute angle command [deg] and max current [mA]/Enabled Subsystem (PID setting) ==
  P : Inport
  I : Inport  Port=2
  D : Inport  Port=3
  Enable : EnablePort
  " x 10^5 " : Gain  Gain=1e5
  Data Type Conversion1 : DataTypeConversion  OutDataTypeStr=uint32  SaturateOnIntegerOverflow=off  RndMeth=Floor
  Data Type Conversion2 : DataTypeConversion  OutDataTypeStr=uint32  SaturateOnIntegerOverflow=off  RndMeth=Floor
  Data Type Conversion3 : DataTypeConversion  OutDataTypeStr=uint32  SaturateOnIntegerOverflow=off  RndMeth=Floor
  I2C Write (0xA0) : arduinolib/I2C Write  I2CModule=0  Mode=Master  SlaveAddress=I2CAddress  SlaveByteOrder=LittleEndian  Direction=Transmitter  RegisterAddressMode=on  RegisterAddress=0xA0  SlaveDataType=uint8  DataLength=1  NoAck=off  RepeatedStart=off  OutputStatus=off  blockPlatform=ARDUINO
  I2C Write (0xA4) : arduinolib/I2C Write  I2CModule=0  Mode=Master  SlaveAddress=I2CAddress  SlaveByteOrder=LittleEndian  Direction=Transmitter  RegisterAddressMode=on  RegisterAddress=0xA4  SlaveDataType=uint8  DataLength=1  NoAck=off  RepeatedStart=off  OutputStatus=off  blockPlatform=ARDUINO
  I2C Write (0xA8) : arduinolib/I2C Write  I2CModule=0  Mode=Master  SlaveAddress=I2CAddress  SlaveByteOrder=LittleEndian  Direction=Transmitter  RegisterAddressMode=on  RegisterAddress=0xA8  SlaveDataType=uint8  DataLength=1  NoAck=off  RepeatedStart=off  OutputStatus=off  blockPlatform=ARDUINO
  x 10^5 : Gain  Gain=1e5
  x 10^7 : Gain  Gain=1e7
  wires:
  P/1 -> x 10^5/1
  I/1 -> x 10^7/1
  D/1 -> " x 10^5 "/1
  Data Type Conversion2/1 -> I2C Write (0xA4)/1
  Data Type Conversion3/1 -> I2C Write (0xA8)/1
  Data Type Conversion1/1 -> I2C Write (0xA0)/1
  x 10^5/1 -> Data Type Conversion1/1
  x 10^7/1 -> Data Type Conversion2/1
  " x 10^5 "/1 -> Data Type Conversion3/1
